simulink model "Stability_Study_QUATERNION111"  (R2019a)
settings: Solver=VariableStepAuto  StartTime=0.0  StopTime=100.0  RelTol=1e-3
libraries: shared6dof x1, aerolibnav x1
settings Model: Creator=thibault  LastModifiedBy=thibault
settings DataIOCC: ReturnWorkspaceOutputs=off
settings DebuggingCC: PregeneratedLibrarySubsystemCodeDiagnostic=none  ArithmeticOperatorsInVariantConditions=warning
settings SFSimCC: SimUseLocalCustomCode=off
settings RTWCC: RTWUseLocalCustomCode=off

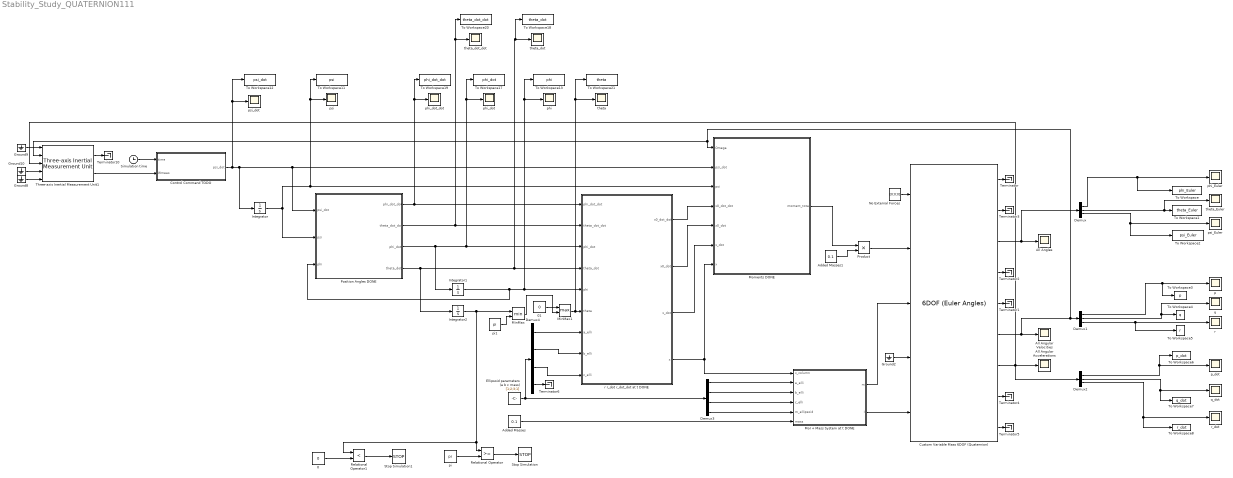
== system Stability_Study_QUATERNION111 ==
  0 : Constant  Value=0
  01 : Constant  Value=0
  Added Masses : Constant  Value=0.1
  Added Masses1 : Constant  Value=0.1
  All Angles : Scope
  All Angular Accelerations : Scope
  All Angular Velocities : Scope
  Control Command TODO : MATLAB Function  TreatAsAtomicUnit=on
  Custom Variable Mass 6DOF (Quaternion) : shared6dof/6DOF (Euler Angles)  units=Metric (MKS)  mtype=Custom Variable  rep=Quaternion  xme_0=[0 0 0]  Vm_0=[0 0 0]  eul_0=[0 0 0]  pm_0=[0 0 1]  mass_0=1.0  mass_e=0.5  mass_f=2.0  inertia=eye(3)  inertia_e=eye(3)  inertia_f=2*eye(3)  k_quat=1.0  vre_flag=off  abi_flag=on  aMode=0  xme_statename=''  Vm_statename=''  eul_statename=''  quat_statename=''  pm_statename=''  mass_statename=''
      settings: SourceProductBaseCode=AE
  Demux : Demux  Outputs=3
  Demux1 : Demux  Outputs=3
  Demux2 : Demux  Outputs=3
  Demux3 : Demux
  Demux4 : Demux
  Ellipsoid parameters (a b c mass) : Constant  Value=[1;2;3;1]  VectorParams1D=off
  Ground{2,8..10} (4 alike) : Ground
  Integrator : Integrator
  Integrator1 : Integrator
  Integrator2 : Integrator
  MinMax : MinMax  Inputs=2
  MinMax1 : MinMax  Function=max  Inputs=2
  MoI + Mass System at t DONE : MATLAB Function  TreatAsAtomicUnit=on
  Moments DONE : MATLAB Function  TreatAsAtomicUnit=on
  No External Forces : Constant  Value=[0;0;0]
  Position Angles DONE : MATLAB Function  TreatAsAtomicUnit=on
  Product : Product
  Relational Operator : RelationalOperator  OutDataTypeStr=boolean  RndMeth=Simplest
  Relational Operator1 : RelationalOperator  Operator=<  OutDataTypeStr=boolean  RndMeth=Simplest
  Simulation time : Clock
  Stop Simulation : Stop
  Stop Simulation1 : Stop
  Terminator{,1..6,10} (8 alike) : Terminator
  Three-axis Inertial Measurement Unit1 : aerolibnav/Three-axis Inertial Measurement Unit  units=Metric (MKS)  imu=[0 0 0]  i_Ts=0  dtype_a=on  w_a=190  z_a=0.707  a_sf_cc=[1 0 0; 0 1 0; 0 0 1]  a_bias=[0 0 0]  a_sat="[-inf  -inf  -inf  inf inf inf]"  dtype_g=on  w_g=190  z_g=0.707  g_sf_cc=[1 0 0; 0 1 0; 0 0 1]  g_bias=[0 0 0]  g_sens=[0 0 0]  g_sat="[-inf  -inf  -inf  inf inf inf]"  i_rand=on  i_seeds=[23093 23094 23095 23096 23097 23098]  i_pow=[0.001 0.001 0.001 0.0001 0.0001 0.0001]
  To Workspace : ToWorkspace  VariableName=phi_Euler  SaveFormat=Timeseries  SampleTime=-1
  To Workspace1 : ToWorkspace  VariableName=theta_Euler  SaveFormat=Timeseries  SampleTime=-1
  To Workspace11 : ToWorkspace  VariableName=psi  SaveFormat=Timeseries  SampleTime=-1
  To Workspace12 : ToWorkspace  VariableName=psi_dot  SaveFormat=Timeseries  SampleTime=-1
  To Workspace13 : ToWorkspace  VariableName=phi  SaveFormat=Timeseries  SampleTime=-1
  To Workspace17 : ToWorkspace  VariableName=phi_dot  SaveFormat=Timeseries  SampleTime=-1
  To Workspace18 : ToWorkspace  VariableName=theta_dot  SaveFormat=Timeseries  SampleTime=-1
  To Workspace19 : ToWorkspace  VariableName=phi_dot_dot  SaveFormat=Timeseries  SampleTime=-1
  To Workspace2 : ToWorkspace  VariableName=psi_Euler  SaveFormat=Timeseries  SampleTime=-1
  To Workspace20 : ToWorkspace  VariableName=theta_dot_dot  SaveFormat=Timeseries  SampleTime=-1
  To Workspace21 : ToWorkspace  VariableName=theta  SaveFormat=Timeseries  SampleTime=-1
  To Workspace3 : ToWorkspace  VariableName=p  SaveFormat=Timeseries  SampleTime=-1
  To Workspace4 : ToWorkspace  VariableName=q  SaveFormat=Timeseries  SampleTime=-1
  To Workspace5 : ToWorkspace  VariableName=r  SaveFormat=Timeseries  SampleTime=-1
  To Workspace6 : ToWorkspace  VariableName=p_dot  SaveFormat=Timeseries  SampleTime=-1
  To Workspace7 : ToWorkspace  VariableName=q_dot  SaveFormat=Timeseries  SampleTime=-1
  To Workspace8 : ToWorkspace  VariableName=r_dot  SaveFormat=Timeseries  SampleTime=-1
  p : Scope
  p_dot : Scope
  phi : Scope
  phi_Euler : Scope
  phi_dot : Scope
  phi_dot_dot : Scope
  pi : Constant  Value=pi
  pi1 : Constant  Value=pi
  psi : Scope
  psi_Euler : Scope
  psi_dot : Scope
  q : Scope
  q_dot : Scope
  r : Scope
  r r_dot r_dot_dot at t DONE : MATLAB Function  TreatAsAtomicUnit=on
  r_dot : Scope
  theta : Scope
  theta_Euler : Scope
  theta_dot : Scope
  theta_dot_dot : Scope
  wires:
  No External Forces/1 -> Custom Variable Mass 6DOF (Quaternion)/1
  Custom Variable Mass 6DOF (Quaternion)/1 -> Terminator/1
  Custom Variable Mass 6DOF (Quaternion)/2 -> Terminator3/1
  Custom Variable Mass 6DOF (Quaternion)/4 -> Terminator2/1
  Custom Variable Mass 6DOF (Quaternion)/5 -> Terminator1/1
  Custom Variable Mass 6DOF (Quaternion)/3 -> Demux/1, All Angles/1
  Demux/1 -> To Workspace/1, phi_Euler/1
  Demux/2 -> To Workspace1/1, theta_Euler/1
  Demux/3 -> To Workspace2/1, psi_Euler/1
  Custom Variable Mass 6DOF (Quaternion)/8 -> Terminator4/1
  Custom Variable Mass 6DOF (Quaternion)/9 -> Terminator5/1
  Custom Variable Mass 6DOF (Quaternion)/6 -> Moments DONE/1(Omega), Three-axis Inertial Measurement Unit1/2, Demux1/1, All Angular Velocities/1
  Demux1/1 -> To Workspace3/1, p/1
  Demux1/2 -> q/1, To Workspace4/1
  Demux1/3 -> To Workspace5/1, r/1
  Demux2/1 -> To Workspace6/1, p_dot/1
  Demux2/2 -> To Workspace7/1, q_dot/1
  Demux2/3 -> To Workspace8/1, r_dot/1
  Custom Variable Mass 6DOF (Quaternion)/7 -> Three-axis Inertial Measurement Unit1/3, Demux2/1, All Angular Accelerations/1
  Ellipsoid parameters (a b c mass)/1 -> Demux3/1, Demux4/1
  MoI + Mass System at t DONE/2(I) -> Custom Variable Mass 6DOF (Quaternion)/5
  r r_dot r_dot_dot at t DONE/4(x) -> Moments DONE/7(x), MoI + Mass System at t DONE/1(x_column)
  Demux3/4 -> MoI + Mass System at t DONE/5(m_ellipsoid)
  Demux3/3 -> MoI + Mass System at t DONE/4(c_elli)
  Demux3/2 -> MoI + Mass System at t DONE/3(b_elli)
  Demux3/1 -> MoI + Mass System at t DONE/2(a_elli)
  Added Masses/1 -> MoI + Mass System at t DONE/6(mass)
  MoI + Mass System at t DONE/1(m) -> Custom Variable Mass 6DOF (Quaternion)/3
  Demux4/4 -> Terminator6/1
  Demux4/3 -> r r_dot r_dot_dot at t DONE/9(c_elli)
  Demux4/2 -> r r_dot r_dot_dot at t DONE/8(b_elli)
  Demux4/1 -> r r_dot r_dot_dot at t DONE/7(a_elli)
  Product/1 -> Custom Variable Mass 6DOF (Quaternion)/2
  Moments DONE/1(moment_total) -> Product/1
  Control Command TODO/1(psi_dot) -> To Workspace12/1, psi_dot/1, Integrator/1, Position Angles DONE/1(psi_dot), Moments DONE/2(psi_dot)
  r r_dot r_dot_dot at t DONE/2(x0_dot) -> Moments DONE/5(x0_dot)
  r r_dot r_dot_dot at t DONE/1(x0_dot_dot) -> Moments DONE/4(x0_dot_dot)
  r r_dot r_dot_dot at t DONE/3(x_dot) -> Moments DONE/6(x_dot)
  Integrator/1 -> To Workspace11/1, psi/1, Moments DONE/3(psi), Position Angles DONE/2(psi)
  Added Masses1/1 -> Product/2
  Ground2/1 -> Custom Variable Mass 6DOF (Quaternion)/4
  Position Angles DONE/1(phi_dot_dot) -> r r_dot r_dot_dot at t DONE/1(phi_dot_dot), To Workspace19/1, phi_dot_dot/1
  Position Angles DONE/2(theta_dot_dot) -> r r_dot r_dot_dot at t DONE/2(theta_dot_dot), theta_dot_dot/1, To Workspace20/1
  Position Angles DONE/3(phi_dot) -> To Workspace17/1, phi_dot/1, r r_dot r_dot_dot at t DONE/3(phi_dot), Integrator1/1
  Position Angles DONE/4(theta_dot) -> Integrator2/1, To Workspace18/1, theta_dot/1, r r_dot r_dot_dot at t DONE/4(theta_dot)
  Integrator1/1 -> Position Angles DONE/3(phi), To Workspace13/1, phi/1, r r_dot r_dot_dot at t DONE/5(phi)
  Integrator2/1 -> MinMax/1, Relational Operator1/1, Relational Operator/1
  Simulation time/1 -> Control Command TODO/1(time)
  Relational Operator/1 -> Stop Simulation/1
  pi/1 -> Relational Operator/2
  0/1 -> Relational Operator1/2
  Relational Operator1/1 -> Stop Simulation1/1
  MinMax1/1 -> To Workspace21/1, theta/1, r r_dot r_dot_dot at t DONE/6(theta)
  MinMax/1 -> MinMax1/2
  01/1 -> MinMax1/1
  pi1/1 -> MinMax/2
  Ground10/1 -> Three-axis Inertial Measurement Unit1/4
  Ground8/1 -> Three-axis Inertial Measurement Unit1/5
  Three-axis Inertial Measurement Unit1/1 -> Terminator10/1
  Ground9/1 -> Three-axis Inertial Measurement Unit1/1
  Three-axis Inertial Measurement Unit1/2 -> Control Command TODO/2(Wmeas)

== matlab function Stability_Study_QUATERNION111/Position Angles DONE ==
  data: psi_dot input; psi input; phi_dot_dot output; theta_dot_dot output; phi_dot output; theta_dot output; phi input
function [phi_dot_dot, theta_dot_dot, phi_dot, theta_dot]=angular_position(psi_dot, psi, phi)

phi_dot=psi(3);                                                       %done
phi_dot_dot=psi_dot(3);                                               %done

posOrneg=0;

if(abs(sin(phi))<0.01)
    posOrneg=sign(psi(2)/cos(phi));                                   %done
else
    posOrneg=sign(-psi(1)/sin(phi));                                  %done
end

theta_dot_dot=posOrneg*sqrt(psi_dot(1)^2+psi_dot(2)^2);               %done
theta_dot=posOrneg*sqrt(psi(1)^2+psi(2)^2);                           %done

end

== matlab function Stability_Study_QUATERNION111/Control Command TODO ==
  data: time input; psi_dot output; Wmeas input
function psi_dot = control_command(time, Wmeas)
t=time;

%psi_dot = [0;0;-exp(-t)];
psi_dot = t*[Wmeas(1);Wmeas(2);Wmeas(3)];
end

== matlab function Stability_Study_QUATERNION111/MoI + Mass System at t DONE ==
  data: m output; x_column input; a_elli input; b_elli input; c_elli input; m_ellipsoid input; I output; mass input
function [m, I] = MoI(x_column, a_elli, b_elli, c_elli, m_ellipsoid, mass)

m=mass+m_ellipsoid; %total mass

a=a_elli;
b=b_elli;
c=c_elli;

x=x_column;

I=0.2*m_ellipsoid*[b^2+c^2 0 0;
               0 a^2+c^2 0;
               0 0 a^2+b^2]+mass*(dot(x,x)*eye(3)-kron(x,x')); 
%assuming x column vector
%this is valid for symetric masses ie mass is the total added mass since
%the formula gives the same result for x and -x
%DONE
end

== matlab function Stability_Study_QUATERNION111/r r_dot r_dot_dot at t DONE ==
  data: phi_dot_dot input; x0_dot_dot output; theta_dot_dot input; phi_dot input; theta_dot input; phi input; theta input; x0_dot output; x_dot output; a_elli input; b_elli input; c_elli input; x output
function [x0_dot_dot,x0_dot,x_dot,x] = radii(phi_dot_dot, theta_dot_dot, phi_dot, theta_dot, phi, theta, a_elli, b_elli, c_elli)

%ellipsoid parmeters
a2 = a_elli^2;
b2 = b_elli^2;
c2 = c_elli^2;

%angles and angular velocities
phidd = phi_dot_dot;
thetadd = theta_dot_dot;
phid = phi_dot;
thetad = theta_dot;

%trigonometric function calculated only once!!
cosp = cos(phi);
sinp = sin(phi);
cos2p = cos(2*phi);
sin2p = sin(2*phi);
cost = cos(theta);
sint = sin(theta);
cos2t = cos(2*theta);
sin2t = sin(2*theta);

%OK done base
base = (cosp^2)*(sint^2)/a2 + (sinp^2)*(sint^2)/b2 + cost^2/c2;

%OK prime done
prime = (cosp^2*sin2t*thetad - sin2p*phid*sint^2)/a2 + (sinp^2*sin2t*thetad + sin2p*phid*sint^2)/b2 - (sin2t*thetad)/c2;

%OK second done
prime_a_dot = (cosp^2*cos2t*2*thetad^2 + cosp^2*sin2t*thetadd - 2*sin2p*phid*sin2t*thetad - 2*cos2p*phid^2*sint^2 - sin2p*phidd*sint^2)/a2; %done
prime_b_dot = (sinp^2*2*cos2t*thetad^2 + sinp^2*sin2t*thetadd + 2*sin2p*phid*sin2t*thetad + 2*cos2p*phid^2*sint^2 + sin2p*phidd*sint^2)/b2; %done
prime_c_dot = -(2*cos2t*thetad^2 + sin2t*thetadd)/c2; %done

second = prime_a_dot + prime_b_dot + prime_c_dot;

r = sqrt(1/base); %done
r_dot = -0.5*r^3*prime; %done
r_dot_dot = 0.75*r^5*prime^2 - 0.5*r^3*second; %done

e_r = [cosp*sint;sinp*sint;cost]; %done
e_phi = [-sinp;cosp;0]; %done
e_theta = [cosp*cost;sinp*cost;-sint]; %done

x = r*e_r; %done
x_dot = r_dot*e_r + r*(phid*sint*e_phi + thetad*e_theta); %done
x0_dot = r_dot*e_r; %done
x0_dot_dot = r_dot_dot*e_r; %done
end

== matlab function Stability_Study_QUATERNION111/Moments DONE ==
  data: Omega input; psi_dot input; psi input; x0_dot_dot input; x0_dot input; x_dot input; x input; moment_total output
function moment_total = moments(Omega, psi_dot, psi, x0_dot_dot,x0_dot, x_dot,x)
%the moment calculated here is per unit of mass need to be multipled by
%added mass

momentJ=-2*(dot(x0_dot,x)*eye(3)-kron(x0_dot,x'))*Omega; %DONE
moment1=(kron(x0_dot,x')-kron(x,x0_dot'))*psi; %DONE
moment2=-(kron(x,cross(x,psi)')+kron(x,cross(x,psi)')')*Omega; %DONE
moment3=-cross(x,x0_dot_dot); %DONE
moment4=-(dot(x,x)*eye(3)-kron(x,x'))*psi_dot - (2*dot(x,x_dot)*eye(3)-kron(x_dot,x')-kron(x,x_dot'))*psi; %DONE

moment_total = momentJ+moment1+moment2+moment3+moment4; %DONE
end
